simulink model "motore"  (R2014a)
settings: Solver=ode45  StartTime=0.0  StopTime=10  RelTol=1e-3
values from neighbouring files (symbols this model uses):
  B = 0.1    [motore_matlab.m]    (also in parameters.m)
  J = 0.01    [motore_matlab.m]    (also in parameters.m)
  kb = 0.01    [motore_matlab.m]    (also in parameters.m)
  kt = 0.01    [motore_matlab.m]    (also in parameters.m)
  Lm = 0.5    [motore_matlab.m]    (also in parameters.m)
  Rm = 1    [motore_matlab.m]    (also in parameters.m)
settings Model: Creator=chiarafoglietta  LastModifiedBy=chiarafoglietta

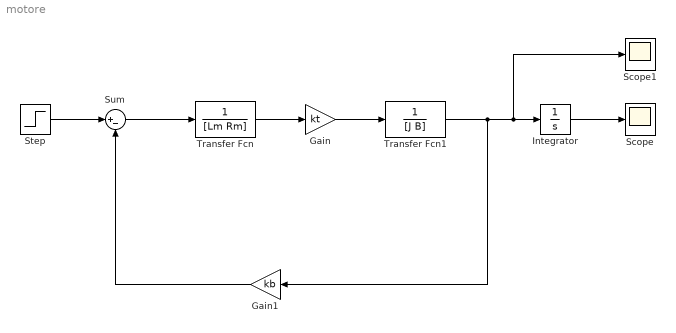
== system motore ==
  Gain : Gain  Gain=kt
  Gain1 : Gain  Gain=kb
  Integrator : Integrator
  Scope : Scope
  Scope1 : Scope
  Step : Step  After=5  SampleTime=0
  Sum : Sum  Inputs=|+-
  Transfer Fcn : TransferFcn  Denominator=[Lm Rm]
  Transfer Fcn1 : TransferFcn  Denominator=[J B]
  wires:
  Sum/1 -> Transfer Fcn/1
  Transfer Fcn/1 -> Gain/1
  Gain/1 -> Transfer Fcn1/1
  Transfer Fcn1/1 -> Gain1/1, Scope1/1, Integrator/1
  Gain1/1 -> Sum/2
  Step/1 -> Sum/1
  Integrator/1 -> Scope/1
